simulink model "model_tugas3"  (R2013a)
settings: Solver=ode15s  StartTime=0.0  StopTime=1.0  RelTol=1e-3
model workspace (MAT data in the model file):
  R1 = 10
  R2 = 10
  R3 = 10
  R4 = 10
  V = 9
libraries: fl_lib x29, nesl_utility x16
settings Model: Creator=SPC LIFE 5  LastModifiedBy=SPC LIFE 5
settings DataIOCC: InspectSignalLogs=on
settings DebuggingCC: SolverPrmCheckMsg=none

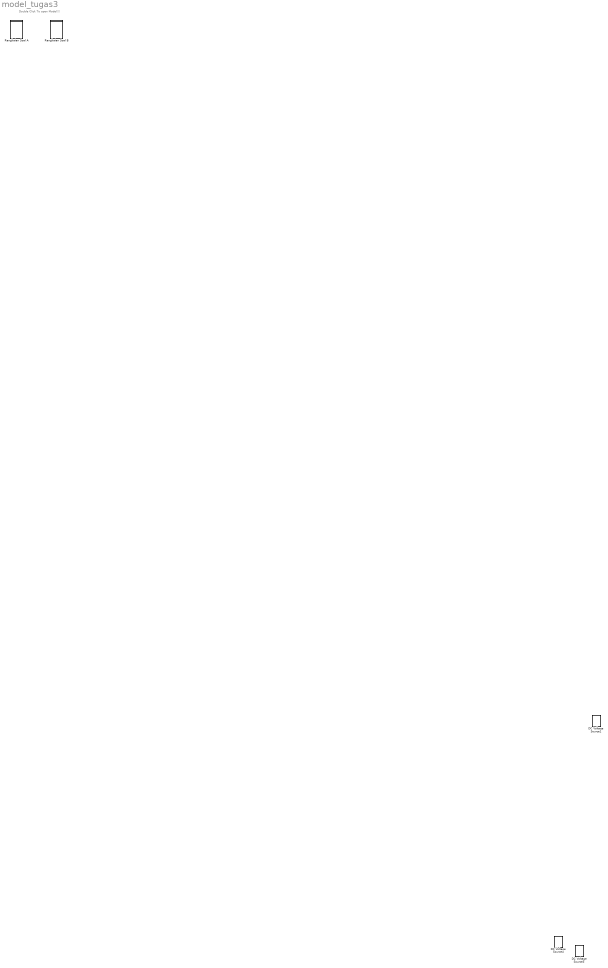
== system model_tugas3 ==
  note: Double Click To open Model!!!
  DC Voltage Source1 : fl_lib/Electrical/Electrical Sources/DC Voltage Source  v0=1 V  i_Log=off  v_Log=off  LocalVarNames=|i|v  LocalVarDescs=|i|v  LocalVarLogging=[0 0]
  DC Voltage Source3 : fl_lib/Electrical/Electrical Sources/DC Voltage Source  v0=1 V  i_Log=off  v_Log=off  LocalVarNames=|i|v  LocalVarDescs=|i|v  LocalVarLogging=[0 0]
  DC Voltage Source4 : fl_lib/Electrical/Electrical Sources/DC Voltage Source  v0=1 V  i_Log=off  v_Log=off  LocalVarNames=|i|v  LocalVarDescs=|i|v  LocalVarLogging=[0 0]
  Rangkaian Soal A : Subsystem
  Rangkaian Soal B : Subsystem

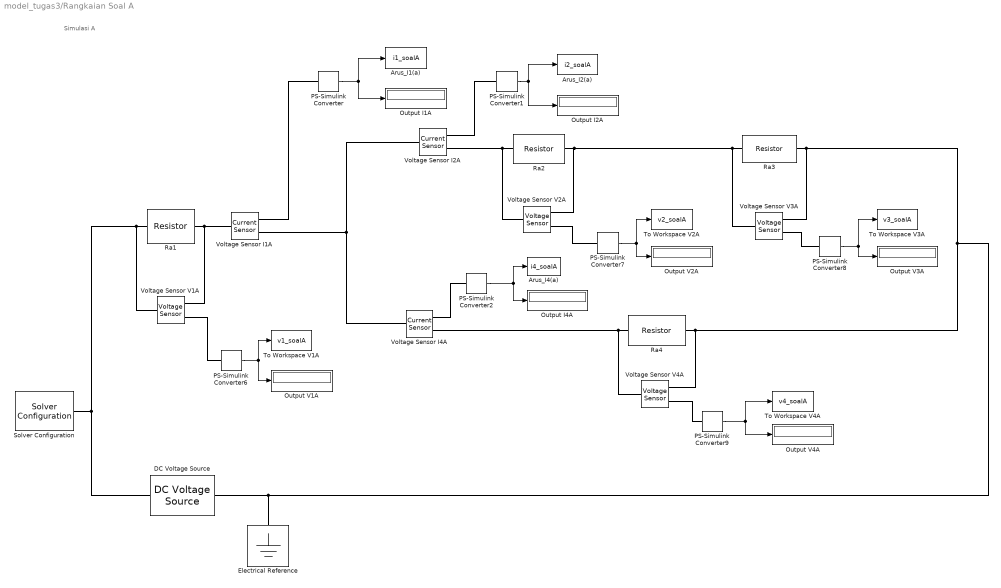
== system model_tugas3/Rangkaian Soal A ==
  note: Simulasi A
  Arus_I1(a) : ToWorkspace  VariableName=i1_soalA  SampleTime=-1
  Arus_I2(a) : ToWorkspace  VariableName=i2_soalA  SampleTime=-1
  Arus_I4(a) : ToWorkspace  VariableName=i4_soalA  SampleTime=-1
  DC Voltage Source : fl_lib/Electrical/Electrical Sources/DC Voltage Source  v0=V V  i_Log=off  v_Log=off  LocalVarNames=|i|v  LocalVarDescs=|i|v  LocalVarLogging=[0 0]
  Electrical Reference : fl_lib/Electrical/Electrical Elements/Electrical Reference  i_Log=off  LocalVarNames=|i  LocalVarDescs=|i  LocalVarLogging=0
  Output I1A : Display
  Output I2A : Display
  Output I4A : Display
  Output V1A : Display
  Output V2A : Display
  Output V3A : Display
  Output V4A : Display
  PS-Simulink Converter{,1..2,6..9} (7 alike) : nesl_utility/PS-Simulink Converter  PhysicalDomain=network_engine_domain  SubClassName=ps_output  LeftPortType=input  RightPortType=output  PseudoPeriodic=off  Frequencies=[]  Unit=1  AffineConversion=off
  Ra1 : fl_lib/Electrical/Electrical Elements/Resistor  R=R1 Ohm  i_Log=off  v_Log=off  LocalVarNames=|i|v  LocalVarDescs=|i|v  LocalVarLogging=[0 0]
  Ra2 : fl_lib/Electrical/Electrical Elements/Resistor  R=R2 Ohm  i_Log=off  v_Log=off  LocalVarNames=|i|v  LocalVarDescs=|i|v  LocalVarLogging=[0 0]
  Ra3 : fl_lib/Electrical/Electrical Elements/Resistor  R=R3 Ohm  i_Log=off  v_Log=off  LocalVarNames=|i|v  LocalVarDescs=|i|v  LocalVarLogging=[0 0]
  Ra4 : fl_lib/Electrical/Electrical Elements/Resistor  R=R4 Ohm  i_Log=off  v_Log=off  LocalVarNames=|i|v  LocalVarDescs=|i|v  LocalVarLogging=[0 0]
  Solver Configuration : nesl_utility/Solver Configuration  PhysicalDomain=network_engine_domain  SubClassName=solver  LeftPortType=input  RightPortType=generic  Accelerate=off  Tones=[]  Harmonics=[]  SimulateNoise=off  Profile=off  UseLocalSampling=off  EnableSwitchedLinearOptims=on  FrequencyDomain=off  UseCCode=off  UseNewInitialization=off  DoDC=off  ResidualTolerance=1e-09  UseLocalSolver=off  LocalSolverChoice=NE_BACKWARD_EULER_ADVANCER  LocalSolverSampleTime=0.001  DoFixedCost=off  MaxNonlinIter=3  MaxModeIter=2  LinearAlgebra=Sparse  DelaysMemoryBudget=1024
  To Workspace V1A : ToWorkspace  VariableName=v1_soalA  SampleTime=-1  SaveFormat=Timeseries
  To Workspace V2A : ToWorkspace  VariableName=v2_soalA  SampleTime=-1  SaveFormat=Timeseries
  To Workspace V3A : ToWorkspace  VariableName=v3_soalA  SampleTime=-1
  To Workspace V4A : ToWorkspace  VariableName=v4_soalA  SampleTime=-1  SaveFormat=Timeseries
  Voltage Sensor I1A : fl_lib/Electrical/Electrical Sensors/Current Sensor  i1_Log=off  v1_Log=off  LocalVarNames=|i1|v1  LocalVarDescs=|i1|v1  LocalVarLogging=[0 0]
  Voltage Sensor I2A : fl_lib/Electrical/Electrical Sensors/Current Sensor  i1_Log=off  v1_Log=off  LocalVarNames=|i1|v1  LocalVarDescs=|i1|v1  LocalVarLogging=[0 0]
  Voltage Sensor I4A : fl_lib/Electrical/Electrical Sensors/Current Sensor  i1_Log=off  v1_Log=off  LocalVarNames=|i1|v1  LocalVarDescs=|i1|v1  LocalVarLogging=[0 0]
  Voltage Sensor V1A : fl_lib/Electrical/Electrical Sensors/Voltage Sensor  i1_Log=off  v1_Log=off  LocalVarNames=|i1|v1  LocalVarDescs=|i1|v1  LocalVarLogging=[0 0]
  Voltage Sensor V2A : fl_lib/Electrical/Electrical Sensors/Voltage Sensor  i1_Log=off  v1_Log=off  LocalVarNames=|i1|v1  LocalVarDescs=|i1|v1  LocalVarLogging=[0 0]
  Voltage Sensor V3A : fl_lib/Electrical/Electrical Sensors/Voltage Sensor  i1_Log=off  v1_Log=off  LocalVarNames=|i1|v1  LocalVarDescs=|i1|v1  LocalVarLogging=[0 0]
  Voltage Sensor V4A : fl_lib/Electrical/Electrical Sensors/Voltage Sensor  i1_Log=off  v1_Log=off  LocalVarNames=|i1|v1  LocalVarDescs=|i1|v1  LocalVarLogging=[0 0]
  wires:
  PS-Simulink Converter8/1 -> Output V3A/1, To Workspace V3A/1
  PS-Simulink Converter2/1 -> Output I4A/1, Arus_I4(a)/1
  PS-Simulink Converter7/1 -> To Workspace V2A/1, Output V2A/1
  PS-Simulink Converter/1 -> Output I1A/1, Arus_I1(a)/1
  PS-Simulink Converter1/1 -> Output I2A/1, Arus_I2(a)/1
  PS-Simulink Converter6/1 -> To Workspace V1A/1, Output V1A/1
  PS-Simulink Converter9/1 -> Output V4A/1, To Workspace V4A/1
  connections:
  DC Voltage Source/LConn1 -- Voltage Sensor V1A/LConn1 -- Ra1/LConn1 -- Solver Configuration/RConn1
  Voltage Sensor V1A/RConn1 -- PS-Simulink Converter6/LConn1
  Voltage Sensor V2A/RConn1 -- PS-Simulink Converter7/LConn1
  Ra2/RConn1 -- Voltage Sensor V3A/LConn1 -- Ra3/LConn1 -- Voltage Sensor V2A/RConn2
  Voltage Sensor I2A/RConn2 -- Ra2/LConn1 -- Voltage Sensor V2A/LConn1
  Voltage Sensor I1A/RConn1 -- PS-Simulink Converter/LConn1
  Voltage Sensor I2A/LConn1 -- Voltage Sensor I4A/LConn1 -- Voltage Sensor I1A/RConn2
  Voltage Sensor V3A/RConn1 -- PS-Simulink Converter8/LConn1
  Ra1/RConn1 -- Voltage Sensor I1A/LConn1 -- Voltage Sensor V1A/RConn2
  Voltage Sensor V4A/RConn1 -- PS-Simulink Converter9/LConn1
  Voltage Sensor I2A/RConn1 -- PS-Simulink Converter1/LConn1
  Voltage Sensor I4A/RConn1 -- PS-Simulink Converter2/LConn1
  Voltage Sensor I4A/RConn2 -- Voltage Sensor V4A/LConn1 -- Ra4/LConn1
  Ra3/RConn1 -- Electrical Reference/LConn1 -- DC Voltage Source/RConn1 -- Voltage Sensor V4A/RConn2 -- Ra4/RConn1 -- Voltage Sensor V3A/RConn2

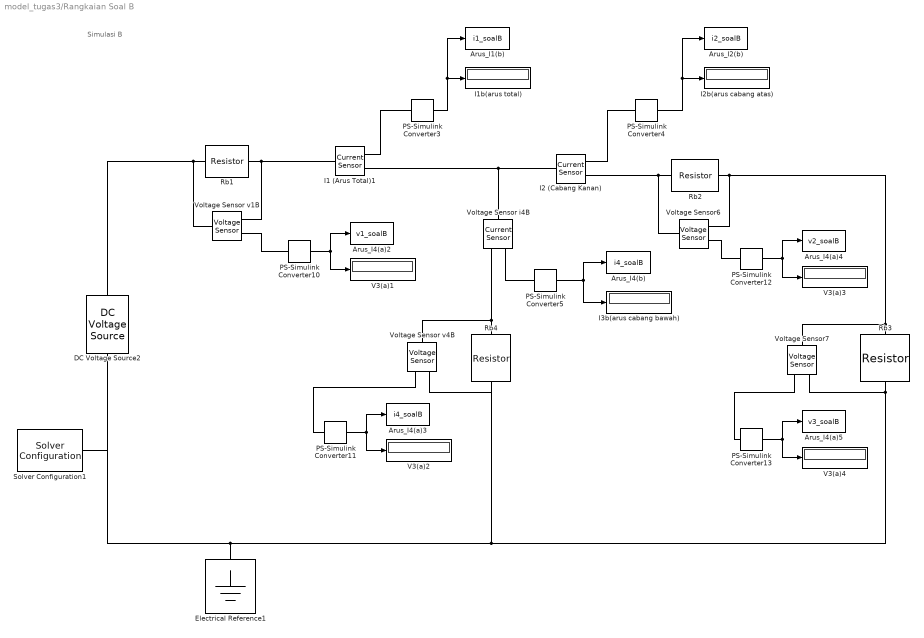
== system model_tugas3/Rangkaian Soal B ==
  note: Simulasi B
  Arus_I1(b) : ToWorkspace  VariableName=i1_soalB  SampleTime=-1
  Arus_I2(b) : ToWorkspace  VariableName=i2_soalB  SampleTime=-1
  Arus_I4(a)2 : ToWorkspace  VariableName=v1_soalB  SampleTime=-1
  Arus_I4(a)3 : ToWorkspace  VariableName=i4_soalB  SampleTime=-1
  Arus_I4(a)4 : ToWorkspace  VariableName=v2_soalB  SampleTime=-1
  Arus_I4(a)5 : ToWorkspace  VariableName=v3_soalB  SampleTime=-1
  Arus_I4(b) : ToWorkspace  VariableName=i4_soalB  SampleTime=-1
  DC Voltage Source2 : fl_lib/Electrical/Electrical Sources/DC Voltage Source  v0=V V  i_Log=off  v_Log=off  LocalVarNames=|i|v  LocalVarDescs=|i|v  LocalVarLogging=[0 0]
  Electrical Reference1 : fl_lib/Electrical/Electrical Elements/Electrical Reference  i_Log=off  LocalVarNames=|i  LocalVarDescs=|i  LocalVarLogging=0
  I1 (Arus Total)1 : fl_lib/Electrical/Electrical Sensors/Current Sensor  i1_Log=off  v1_Log=off  LocalVarNames=|i1|v1  LocalVarDescs=|i1|v1  LocalVarLogging=[0 0]
  I1b(arus total) : Display
  I2 (Cabang Kanan) : fl_lib/Electrical/Electrical Sensors/Current Sensor  i1_Log=off  v1_Log=off  LocalVarNames=|i1|v1  LocalVarDescs=|i1|v1  LocalVarLogging=[0 0]
  I2b(arus cabang atas) : Display
  I3b(arus cabang bawah) : Display
  PS-Simulink Converter{3..5,10..13} (7 alike) : nesl_utility/PS-Simulink Converter  PhysicalDomain=network_engine_domain  SubClassName=ps_output  LeftPortType=input  RightPortType=output  PseudoPeriodic=off  Frequencies=[]  Unit=1  AffineConversion=off
  Rb1 : fl_lib/Electrical/Electrical Elements/Resistor  R=R1 Ohm  i_Log=off  v_Log=off  LocalVarNames=|i|v  LocalVarDescs=|i|v  LocalVarLogging=[0 0]
  Rb2 : fl_lib/Electrical/Electrical Elements/Resistor  R=R2 Ohm  i_Log=off  v_Log=off  LocalVarNames=|i|v  LocalVarDescs=|i|v  LocalVarLogging=[0 0]
  Rb3 : fl_lib/Electrical/Electrical Elements/Resistor  R=R3 Ohm  i_Log=off  v_Log=off  LocalVarNames=|i|v  LocalVarDescs=|i|v  LocalVarLogging=[0 0]
  Rb4 : fl_lib/Electrical/Electrical Elements/Resistor  R=R4 Ohm  i_Log=off  v_Log=off  LocalVarNames=|i|v  LocalVarDescs=|i|v  LocalVarLogging=[0 0]
  Solver Configuration1 : nesl_utility/Solver Configuration  PhysicalDomain=network_engine_domain  SubClassName=solver  LeftPortType=input  RightPortType=generic  Accelerate=off  Tones=[]  Harmonics=[]  SimulateNoise=off  Profile=off  UseLocalSampling=off  EnableSwitchedLinearOptims=on  FrequencyDomain=off  UseCCode=off  UseNewInitialization=off  DoDC=off  ResidualTolerance=1e-09  UseLocalSolver=off  LocalSolverChoice=NE_BACKWARD_EULER_ADVANCER  LocalSolverSampleTime=0.001  DoFixedCost=off  MaxNonlinIter=3  MaxModeIter=2  LinearAlgebra=Sparse  DelaysMemoryBudget=1024
  V3(a){1..4} (4 alike) : Display
  Voltage Sensor i4B : fl_lib/Electrical/Electrical Sensors/Current Sensor  i1_Log=off  v1_Log=off  LocalVarNames=|i1|v1  LocalVarDescs=|i1|v1  LocalVarLogging=[0 0]
  Voltage Sensor v1B : fl_lib/Electrical/Electrical Sensors/Voltage Sensor  i1_Log=off  v1_Log=off  LocalVarNames=|i1|v1  LocalVarDescs=|i1|v1  LocalVarLogging=[0 0]
  Voltage Sensor v4B : fl_lib/Electrical/Electrical Sensors/Voltage Sensor  i1_Log=off  v1_Log=off  LocalVarNames=|i1|v1  LocalVarDescs=|i1|v1  LocalVarLogging=[0 0]
  Voltage Sensor6 : fl_lib/Electrical/Electrical Sensors/Voltage Sensor  i1_Log=off  v1_Log=off  LocalVarNames=|i1|v1  LocalVarDescs=|i1|v1  LocalVarLogging=[0 0]
  Voltage Sensor7 : fl_lib/Electrical/Electrical Sensors/Voltage Sensor  i1_Log=off  v1_Log=off  LocalVarNames=|i1|v1  LocalVarDescs=|i1|v1  LocalVarLogging=[0 0]
  wires:
  PS-Simulink Converter11/1 -> Arus_I4(a)3/1, V3(a)2/1
  PS-Simulink Converter12/1 -> Arus_I4(a)4/1, V3(a)3/1
  PS-Simulink Converter10/1 -> Arus_I4(a)2/1, V3(a)1/1
  PS-Simulink Converter13/1 -> Arus_I4(a)5/1, V3(a)4/1
  PS-Simulink Converter5/1 -> Arus_I4(b)/1, I3b(arus cabang bawah)/1
  PS-Simulink Converter3/1 -> Arus_I1(b)/1, I1b(arus total)/1
  PS-Simulink Converter4/1 -> I2b(arus cabang atas)/1, Arus_I2(b)/1
  connections:
  Voltage Sensor6/RConn1 -- PS-Simulink Converter12/LConn1
  Voltage Sensor v4B/RConn1 -- PS-Simulink Converter11/LConn1
  Voltage Sensor v1B/RConn1 -- PS-Simulink Converter10/LConn1
  Voltage Sensor7/RConn1 -- PS-Simulink Converter13/LConn1
  Electrical Reference1/LConn1 -- DC Voltage Source2/RConn1 -- Solver Configuration1/RConn1 -- Rb4/RConn1 -- Voltage Sensor v4B/RConn2 -- Voltage Sensor7/RConn2 -- Rb3/RConn1
  DC Voltage Source2/LConn1 -- Voltage Sensor v1B/LConn1 -- Rb1/LConn1
  I1 (Arus Total)1/RConn2 -- Voltage Sensor i4B/LConn1 -- I2 (Cabang Kanan)/LConn1
  Voltage Sensor i4B/RConn1 -- PS-Simulink Converter5/LConn1
  I2 (Cabang Kanan)/RConn1 -- PS-Simulink Converter4/LConn1
  I1 (Arus Total)1/RConn1 -- PS-Simulink Converter3/LConn1
  I2 (Cabang Kanan)/RConn2 -- Voltage Sensor6/LConn1 -- Rb2/LConn1
  Rb2/RConn1 -- Voltage Sensor6/RConn2 -- Voltage Sensor7/LConn1 -- Rb3/LConn1
  Rb4/LConn1 -- Voltage Sensor v4B/LConn1 -- Voltage Sensor i4B/RConn2
  I1 (Arus Total)1/LConn1 -- Rb1/RConn1 -- Voltage Sensor v1B/RConn2
